simulink model "PMSM_DPCC_NLESO_MRAS"  (R2022a)
settings: Solver=FixedStepDiscrete  StartTime=0.0  StopTime=2  FixedStep=Ts  RelTol=1e-3
InitFcn:
  | Ts = 5e-7;%仿真步长
  | Tpwm = 1e-4;%开关周期
  | Tsample = Tpwm/1;%采样周期/控制周期
  | Tspeed = Tsample;%转速采样周期
  | Pn = 4;%电机极对数
  | Ls = 8.5e-3;%定子电感，采用隐极的，Ld=Lq=Ls
  | Rs = 3;%定子电阻
  | flux = 0.1688;%永磁体磁链
  | Vdc = 311;%直流母线电压
  | iqmax = 20;%额定电流
  | J = 5e-3;%转动惯量
  | B = 2.5e-3;%阻尼系数
  | n_init = 0;%初始转速
  | 
  | %这是DSP内部的控制器参数
  | Ls1 = 1*Ls;%电感参数设置为实际电感
  | Ld1 = Ls1;
  | Lq1 = Ls1;
  | Rs1 = 1*Rs;%电阻参数设置为实际电阻
  | flux1 =1*flux;%磁链参数设置为实际磁链
undefined symbols (not defined in the file): DiscIntNeverNeededParam, magnitude
libraries: simulink x9, slpidlib x2, spsDCVoltageSourceLib x1, spsPermanentMagnetSynchronousMachineLib x1, spsUniversalBridgeLib x1, spspowerguiLib x1
(part 1 of 2)
settings Model: SimulationMode=accelerator  Creator=admin  LastModifiedBy=肖思睿
settings SolverCC: AlgebraicLoopSolver=TrustRegion
settings DataIOCC: ReturnWorkspaceOutputs=off
settings DebuggingCC: UnconnectedInputMsg=warning  UnconnectedOutputMsg=warning  UnconnectedLineMsg=warning  SFMachineParentedDataDiag=warning  ArithmeticOperatorsInVariantConditions=warning
settings SFSimCC: CustomCodeUndefinedFunction=UseInterfaceOnly
settings RTWCC: DLArmComputeVersion=19.05

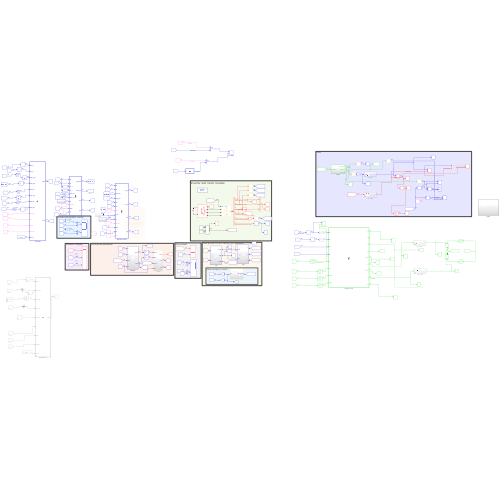
[thumbnail: Simulink's stored preview of the top-level diagram]
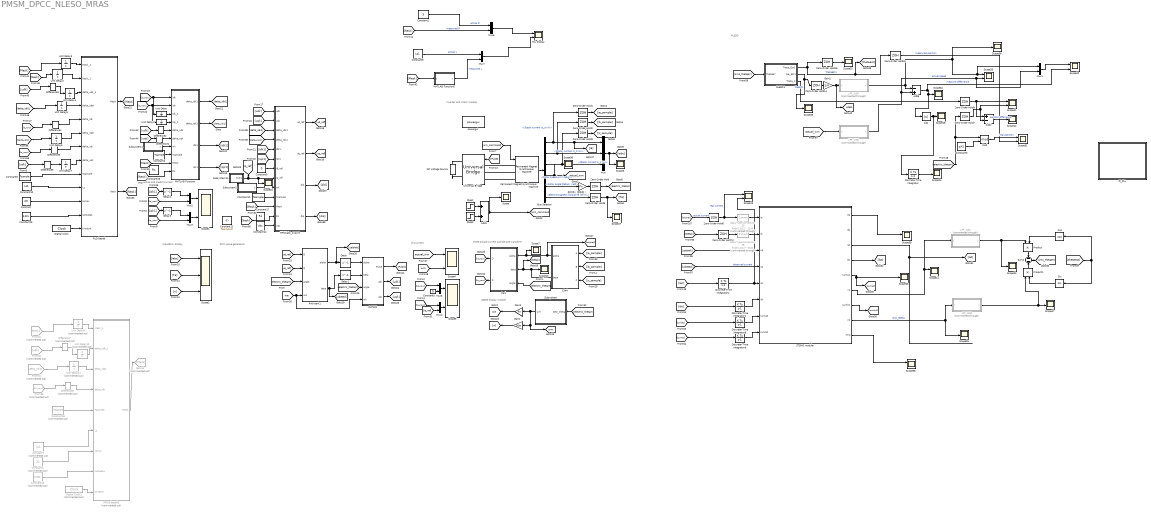
== system PMSM_DPCC_NLESO_MRAS ==
  note: NLESO
  note: PWM pulse generation
  note: Waveform display
  note: actual and predict current
  note: Inverter and motor module
  note: d-q current
  note: three phrase current sample and transform
  note: Speed display module
  Abs : Abs  SaturateOnIntegerOverflow=off
  Add1 : Sum
  Add2 : Sum  Inputs=+-
  Add5 : Sum  Inputs=-+
  Anti-park1 : Subsystem
  Bus Selector : BusSelector  OutputSignals=Stator current is_a (A),Stator current is_b (A),Stator current is_c (A),Rotor speed wm (rad/s),Rotor angle thetam (rad),Electromagnetic torque Te (N*m)
  Clark : Subsystem
  Constant : Constant  Value=20
  Constant1 : Constant  Value=3
  Constant10 : Constant  Value=Ls1
  Constant11 : Constant  Value=Tsample
  Constant12 : Constant  Value=Tpwm/(Ls)
  Constant13 : Constant  Commented=on  Value=0.001
  Constant14 : Constant  Value=Vdc
  Constant15 : Constant  Value=0.001
  Constant16 : Constant  Value=Rs
  Constant17 : Constant  Value=Rs
  Constant18 : Constant  Commented=on  Value=Tsample
  Constant2 : Constant  Value=Tsample
  Constant3 : Constant  Value=pi*2  OutDataTypeStr=double
  Constant4 : Constant  Commented=on  Value=20
  Constant5 : Constant  Value=0
  Constant6 : Constant  Value=Tsample
  Constant7 : Constant  Commented=on  Value=Ls1
  Constant8 : Constant  Value=Ls1
  Constant9 : Constant  Value=0
  Cos : Trigonometry  Operator=cos
  DC Voltage Source : spsDCVoltageSourceLib/DC Voltage Source  Amplitude=Vdc  Measurements=None
  Data Type Conversion25 : DataTypeConversion  Commented=through  OutDataTypeStr=fixdt(1,16,2^-13,0)  SaturateOnIntegerOverflow=off  RndMeth=Floor
  Data Type Conversion26 : DataTypeConversion  Commented=through  OutDataTypeStr=fixdt(1,16,2^-13,0)  SaturateOnIntegerOverflow=off  RndMeth=Floor
  Delay{,1..3} (4 alike) : Delay  DelayLength=1
  Difference{1..6} (6 alike) : simulink/Discrete/Difference  ICPrevInput=0.0  OutMin=[]  OutMax=[]  OutDataType=fixdt(1, 16)  OutScaling=2^-10  DoSatur=off
  Difference7 : simulink/Discrete/Difference  Commented=on  ICPrevInput=0.0  OutMin=[]  OutMax=[]  OutDataType=fixdt(1, 16)  OutScaling=2^-10  DoSatur=off
  Difference8 : simulink/Discrete/Difference  Commented=on  ICPrevInput=0.0  OutMin=[]  OutMax=[]  OutDataType=fixdt(1, 16)  OutScaling=2^-10  DoSatur=off
  Digital Clock : DigitalClock  SampleTime=1e-4
  Digital Clock1 : DigitalClock  Commented=on  SampleTime=1e-4
  Discrete-Time Integrator : DiscreteIntegrator  SampleTime=-1  ICPrevOutput=DiscIntNeverNeededParam  ICPrevScaledInput=DiscIntNeverNeededParam
  Discrete-Time Integrator1 : DiscreteIntegrator  SampleTime=1e-6  ICPrevOutput=DiscIntNeverNeededParam  ICPrevScaledInput=DiscIntNeverNeededParam
  Discrete-Time Integrator2 : DiscreteIntegrator  SampleTime=1e-6  ICPrevOutput=DiscIntNeverNeededParam  ICPrevScaledInput=DiscIntNeverNeededParam
  Discrete-Time Integrator8 : DiscreteIntegrator  gainval=512  SampleTime=1e-6  ICPrevOutput=DiscIntNeverNeededParam  ICPrevScaledInput=DiscIntNeverNeededParam
  Discrete-Time Integrator9 : DiscreteIntegrator  gainval=512  SampleTime=1e-6  ICPrevOutput=DiscIntNeverNeededParam  ICPrevScaledInput=DiscIntNeverNeededParam
  From15 : From  Commented=on  GotoTag=Mesk
  From16 : From  Commented=on  GotoTag=udk
  From34 : From  Commented=on  GotoTag=delta_idk1
  From35 : From  Commented=on  GotoTag=id_now
  Gain1 : Gain  Gain=30/pi
  Gain2 : Gain  Gain=1/4
  Gain3 : Gain  Gain=Pn
  Goto14 : Goto  Commented=on  GotoTag=Mesk
  LPF_WE1 : Subsystem  Commented=through
  LPF_WE2 : Subsystem  Commented=through
  LPF_WE4 : Subsystem  Commented=through
  LPF_WE6 : Subsystem  Commented=through
  MATLAB Function : MATLAB Function  TreatAsAtomicUnit=on
  MATLAB Function5 : MATLAB Function  TreatAsAtomicUnit=on
  MPCCabc_svpwm : MATLAB Function  TreatAsAtomicUnit=on
  MRAS-based1 : MATLAB Function  Commented=on  TreatAsAtomicUnit=on
  Mod : Math  Operator=mod
  Mux : Mux  Inputs=3
  Mux{1..7} (7 alike) : Mux  Inputs=2
  NLESO1 : Subsystem
  PI_PLL : Subsystem
  "Park " : Subsystem
  Permanent Magnet Synchronous Machine : spsPermanentMagnetSynchronousMachineLib/Permanent Magnet Synchronous Machine  NbPhases=3  FluxDistribution=Sinusoidal  RotorType=Round  MechanicalLoad=Torque Tm  PresetModel=No  ShowDetailedParameters=on  MeasurementBus=off  Resistance=Rs  Inductance=8.5e-3  dqInductances=[0.0009262 0.001024]  La=Ls  MachineConstant=Flux linkage established by magnets (V.s)  Flux=flux  VoltageCst=122.4677  TorqueCst=1.0128  Flat=120  Mechanical=[J B Pn 0]  PolePairs=4  InitialConditions=[n_init/60*2*pi,0, 0,0]  InitialConditions5ph=[0 0 0 0 0 0]  RefAngle=Aligned with phase A axis (original Park)  IterativeDiscreteModel=Trapezoidal non iterative  TsBlock=-1  TsPowergui=0
  Product : Product
  Product1 : Product
  R/L display : Scope  NumInputPorts=2
  RLS-based : MATLAB Function  TreatAsAtomicUnit=on
  STSMO module : MATLAB Function  TreatAsAtomicUnit=on
  SVPWM : Subsystem
  Scope{,3,7,10,12,15..17,23..24,26..28,30,32,34..36} (18 alike) : Scope
  Scope{1,4..5,11,13..14,20,31,33,39,56} (11 alike) : Scope  NumInputPorts=2
  Scope2 : Scope  NumInputPorts=3
  Sin : Trigonometry
  Step2 : Step  Time=0  After=0.1  SampleTime=0
  Step3 : Step  After=2.4  SampleTime=0
  Subsystem : Subsystem
  Subsystem1 : Subsystem
  Subsystem11 : Subsystem
  Subsystem2 : Subsystem
  Sum2 : Sum  Inputs=-|-
  Unit Delay : UnitDelay  SampleTime=-1  HasFrameUpgradeWarning=on
  Unit Delay1 : UnitDelay  SampleTime=-1  HasFrameUpgradeWarning=on
  Unit Delay10 : UnitDelay  Commented=on  SampleTime=Tsample  HasFrameUpgradeWarning=on
  Unit Delay11 : UnitDelay  Commented=on  SampleTime=Tsample  HasFrameUpgradeWarning=on
  Unit Delay2 : UnitDelay  InitialCondition=Rs/2  SampleTime=Tsample  HasFrameUpgradeWarning=on
  Unit Delay3 : UnitDelay  InitialCondition=Tpwm/(Ls)  SampleTime=Tsample  HasFrameUpgradeWarning=on
  Unit Delay{4..7} (4 alike) : UnitDelay  SampleTime=Tsample  HasFrameUpgradeWarning=on
  Unit Delay9 : UnitDelay  Commented=on  InitialCondition=Tpwm/(Ls)  SampleTime=Tsample  HasFrameUpgradeWarning=on
  Universal Bridge : spsUniversalBridgeLib/Universal Bridge  Arms=3  SnubberResistance=1e5  SnubberCapacitance=inf  Device=IGBT / Diodes  Ron=1e-3  Lon=0  ForwardVoltages="[  0  0  ]"  ForwardVoltage=0  GTOparameters=[ 10e-6 , 20e-6 ]  IGBTparameters=[ 1e-6 , 2e-6 ]  Measurements=None  Measurements_2=None  converterType=Rectifier
  Zero-Order Hold{,1..3,5} (5 alike) : ZeroOrderHold  SampleTime=Tsample
  Zero-Order Hold{6..7,9..10,14..16} (7 alike) : ZeroOrderHold  SampleTime=1e-4
  powergui : spspowerguiLib/powergui  Priority=1  SimulationMode=Discrete  SampleTime=Ts  frequency=60  Iterations=50  frequencyindice=0  Pbase=100e6  ErrMax=1e-4  UnitsV=kV  UnitsW=MW  buscounter=0  FunctionMessages=off  echomessages=off  EnableUseOfTLC=off  CurrentSourceSwitches=off  DisableSnubberDevices=off  DisableRonSwitches=off  DisableVfSwitches=off  DisplayEquations=off  AutomaticDiscreteSolvers=off  SolverType=Tustin/Backward Euler (TBE)  Interpol=off  ExternalGateDelay=off  methode=off  Ts=100  x0status=blocks  SPID=off  SwTol=0  HookPort=off  NonlinearTolerance=1e-4  nMaxIteration=100  ContinueOnMaxIteration=off  RestoreLinks=warning  ResistiveCurrentMeasurement=off  Frange=[0:2:500]  Ylog=off  Xlog=on  ShowGrid=off  save=off  variable=ZData  structure=IDPCC_MRAS_IA  ZoomFFT=off  StartTime=0  cycles=24  DisplayStyle=1  fundamental=60  FreqAxis=off  MaxFrequency=20000  frequencyindicesteady=1  RmsSteady=1  display=off
  极对数（电角度） : Gain  Gain=Pn
  tag scope: actual_wm=global, wEst=global, we=global, wm=global
  wires:
  Anti-park1/1(alpha) -> [ualphak], Delay/1
  Anti-park1/2(beta) -> Delay1/1, [ubetak]
  [electric_thetam] -> Anti-park1/3(angle)
  Delay/1 -> SVPWM/1(alpha)
  Delay1/1 -> SVPWM/2(beta)
  SVPWM/1(Pulse) -> [Pulse]
  Constant2/1 -> MATLAB Function/8(Tsample)
  [udk] -> Difference2/1
  Difference1/1 -> MATLAB Function/6(delta_uqk)
  Difference2/1 -> MATLAB Function/5(delta_udk)
  Constant14/1 -> MPCCabc_svpwm/13(Vdc)
  [ud_ref] -> Anti-park1/1(D)
  [uq_ref] -> Anti-park1/2(Q)
  [electric_thetam] -> SVPWM/3(angle)
  [iabc] -> Scope2/1
  [n] -> Scope2/3
  [Te] -> Scope2/2
  [idk1] -> Delay2/1
  Mux2/1 -> Scope1/1
  [iqk1] -> Delay3/1
  [id_now] -> Mux2/2
  Mux3/1 -> Scope1/2
  Delay2/1 -> Mux2/1
  [iq_now] -> Mux3/2
  Delay3/1 -> Mux3/1
  MPCCabc_svpwm/1(ud_ref) -> [ud_ref]
  MPCCabc_svpwm/2(uq_ref) -> [uq_ref]
  SVPWM/2(udk) -> [udk]
  SVPWM/3(uqk) -> [uqk]
  Zero-Order Hold3/1 -> [ic_sample]
  Permanent Magnet Synchronous Machine/1 -> Bus Selector/1
  Bus Selector/3 -> Mux/3, Zero-Order Hold3/1  "<Stator current is_c (A)>"
  Bus Selector/2 -> Mux/2, Zero-Order Hold2/1  "<Stator current is_b (A)>"
  极对数（电角度）/1 -> Zero-Order Hold/1
  Bus Selector/5 -> 极对数（电角度）/1  "<Rotor angle thetam (rad)>"
  Bus Selector/4 -> Scope30/1, [actual_wm]  "<Rotor speed wm (rad/s)>"
  Zero-Order Hold5/1 -> Scope27/1, [Te]
  Zero-Order Hold1/1 -> [ia_sample]
  Mux/1 -> Scope3/1, [iabc]
  Bus Selector/6 -> Zero-Order Hold5/1  "<Electromagnetic torque Te (N*m)>"
  [Pulse] -> Universal Bridge/1
  Zero-Order Hold2/1 -> [ib_sample]
  Bus Selector/1 -> [ia], Mux/1, Zero-Order Hold1/1  "<Stator current is_a (A)>"
  "Park "/1(D) -> [id_now]
  Clark/2(beta) -> [ibetak], "Park "/2(beta), Scope10/1
  Gain3/1 -> [we]
  [ia_sample] -> Clark/1(A)
  Gain1/1 -> [n]
  [electric_thetam] -> Subsystem/1(elec_theta)
  "Park "/2(Q) -> [iq_now]
  [ic_sample] -> Clark/3(C)
  Clark/1(alpha) -> [ialphak], Scope7/1, "Park "/1(alpha)
  Subsystem/1(wm) -> [wm], Gain1/1, Gain3/1
  [electric_thetam] -> "Park "/3(angle)
  Mux5/1 -> Scope5/1
  Constant5/1 -> Mux5/2
  [id_now] -> Mux5/1
  [iq_now] -> Mux4/1
  [iq_ref] -> Mux4/2
  [ib_sample] -> Clark/2(B)
  [wm] -> Scope4/2
  Mux4/1 -> Scope5/2
  [actual_wm] -> Scope4/1
  [we] -> Anti-park1/4(we), SVPWM/4(wk)
  Step2/1 -> Add1/1
  Add1/1 -> Scope/1, [wm_command]
  Step3/1 -> Add1/2
  [id_now] -> Unit Delay/1, MATLAB Function/1(idk)
  [iq_now] -> Unit Delay1/1, MATLAB Function/2(iqk)
  Constant11/1 -> MPCCabc_svpwm/10(Tsample)
  Constant9/1 -> MPCCabc_svpwm/7(id_ref)
  Unit Delay/1 -> MATLAB Function/3(idk_1)
  Unit Delay1/1 -> MATLAB Function/4(iqk_1)
  MATLAB Function/4(iqk1) -> [iqk1]
  MATLAB Function/3(idk1) -> [idk1]
  [iqk1] -> MPCCabc_svpwm/6(iqk1)
  [idk1] -> MPCCabc_svpwm/5(idk1)
  MATLAB Function/2(delta_iqk1) -> [delta_iqk1]
  MATLAB Function/1(delta_idk1) -> [delta_idk1]
  [delta_idk1] -> MPCCabc_svpwm/3(delta_idk1)
  [delta_iqk1] -> MPCCabc_svpwm/4(delta_iqk1)
  [udk] -> MPCCabc_svpwm/1(udk)
  [uqk] -> MPCCabc_svpwm/2(uqk)
  Unit Delay3/1 -> RLS-based/1(Mesk_1)
  [Mesk] -> Unit Delay3/1
  [uqk] -> Difference1/1
  [udk] -> Difference3/1
  Unit Delay4/1 -> RLS-based/3(delta_udk_1)
  Difference3/1 -> Unit Delay4/1
  Unit Delay5/1 -> RLS-based/4(delta_idpk)
  [delta_idk1] -> Unit Delay5/1
  [id_now] -> Difference4/1
  Difference4/1 -> RLS-based/5(delta_idk)
  Constant6/1 -> RLS-based/9(Tsample)
  Constant10/1 -> RLS-based/10(Ls)
  Constant/1 -> RLS-based/11(iqmax)
  Constant15/1 -> RLS-based/12(lanbuda1)
  Constant8/1 -> Mux7/1  "actual L"
  [wm_command] -> Permanent Magnet Synchronous Machine/1
  [Mesk] -> MATLAB Function5/1(u)
  Discrete-Time Integrator9/1 -> STSMO module/8(sumb0)
  STSMO module/4(ibt) -> [ibt]
  STSMO module/7(sumb1) -> [sumb1]
  Product1/1 -> Sum2/2
  [ialphak] -> Zero-Order Hold6/1  "actual current"
  [thetaest] -> Cos/1, Sin/1
  Zero-Order Hold10/1 -> Data Type Conversion26/1
  Cos/1 -> Product/2
  Discrete-Time Integrator2/1 -> Scope13/2, STSMO module/5(ial)  "observed current"
  Discrete-Time Integrator8/1 -> STSMO module/7(suma0)
  [ibetak] -> Zero-Order Hold10/1
  Sin/1 -> Product1/2
  STSMO module/3(iat) -> [iat]
  STSMO module/5(suma1) -> [suma1], Scope28/1
  Sum2/1 -> [smo_thetaerr]
  LPF_WE2/1(y) -> Product1/1, Scope17/1
  Discrete-Time Integrator1/1 -> STSMO module/6(ibl)
  Product/1 -> Sum2/1
  Zero-Order Hold/1 -> [electric_thetam]
  LPF_WE1/1(y) -> Product/1, Scope23/1
  Digital Clock/1 -> RLS-based/13(timecnt)
  RLS-based/1(Mesk) -> [Mesk]
  STSMO module/8(x2) -> Scope26/1, LPF_WE2/1(x)  "Obs_Ebeta"
  STSMO module/6(x1) -> Scope14/1, LPF_WE1/1(x)
  Subsystem11/1(Out1) -> Scope15/1, MPCCabc_svpwm/8(iq_ref), [iq_ref]
  MPCCabc_svpwm/4(diq) -> [diq]
  MPCCabc_svpwm/3(did) -> [did]
  STSMO module/9(tmp) -> Scope56/1
  STSMO module/1(ea) -> Scope39/1
  Data Type Conversion25/1 -> STSMO module/1(ia)
  Data Type Conversion26/1 -> STSMO module/2(ib)
  [ualphak] -> STSMO module/3(ua)
  [ubetak] -> STSMO module/4(ub)
  [suma1] -> Discrete-Time Integrator8/1
  [sumb1] -> Discrete-Time Integrator9/1
  [iat] -> Discrete-Time Integrator2/1
  [ibt] -> Discrete-Time Integrator1/1
  Subsystem2/1(y) -> MPCCabc_svpwm/9(wk)
  Subsystem1/1(y) -> MATLAB Function/7(wk)
  [Mesk] -> MATLAB Function/9(Mesk)
  [Mesk] -> MPCCabc_svpwm/11(Mesk)
  Zero-Order Hold6/1 -> Scope13/1, Data Type Conversion25/1  "real current"
  RLS-based/2(Nesk) -> [Nesk]
  [Nesk] -> Unit Delay2/1
  Unit Delay2/1 -> RLS-based/2(Nesk_1)
  Unit Delay6/1 -> RLS-based/6(delta_iqpk)
  [delta_iqk1] -> Unit Delay6/1
  [iq_now] -> Difference5/1
  Difference5/1 -> RLS-based/7(delta_iqk)
  [Nesk] -> MATLAB Function/10(Rs)
  [Nesk] -> MPCCabc_svpwm/12(Rs)
  [udk] -> Difference6/1
  Difference6/1 -> Unit Delay7/1
  Unit Delay7/1 -> RLS-based/8(delta_uqk)
  Constant1/1 -> Mux6/1  "actual R"
  [Nesk] -> Mux6/2  "measured R"
  MATLAB Function5/1(y) -> Mux7/2  "measured L"
  Mux6/1 -> R/L display/1
  Mux7/1 -> R/L display/2
  [actual_wm] -> LPF_WE6/1(x)
  Discrete-Time Integrator/1 -> Scope24/1
  Gain2/1 -> [wEst], LPF_WE4/1(x)
  [smo_thetaerr] -> NLESO1/1(ThetaErr)
  Zero-Order Hold7/1 -> Scope11/2, Add2/2
  Abs/1 -> Scope16/1, Discrete-Time Integrator/1
  LPF_WE4/1(y) -> Add5/1, Mux1/1, Scope33/1, Scope36/1
  NLESO1/3(Theta_2) -> Zero-Order Hold9/1
  Zero-Order Hold14/1 -> Gain2/1
  Constant3/1 -> Mod/2
  NLESO1/2(We_Est1) -> Scope35/1, Zero-Order Hold14/1  "WeEst1"
  Add5/1 -> Scope20/2, Abs/1, Scope34/1  "measure differrence"
  Zero-Order Hold9/1 -> Add2/1, Scope11/1
  Zero-Order Hold15/1 -> Scope31/2  "measured position"
  NLESO1/1(Theta_Est1) -> Zero-Order Hold16/1, Zero-Order Hold15/1, [thetaest]  "ThetaEst1"
  Mod/1 -> Scope31/1  "real position"
  Mux1/1 -> Scope20/1
  LPF_WE6/1(y) -> Mux1/2, Scope33/2, Add5/2  "actual speed"
  Zero-Order Hold16/1 -> Scope32/1
  [electric_thetam] -> Zero-Order Hold7/1, Mod/1
  Add2/1 -> Scope12/1  "position differrence"
  From15/1 -> Unit Delay9/1
  Constant18/1 -> MRAS-based1/5(Tsample)
  From16/1 -> Difference7/1
  Constant4/1 -> MRAS-based1/7(iqmax)
  Constant13/1 -> MRAS-based1/8(lanbuda1)
  Unit Delay9/1 -> MRAS-based1/1(Mesk_1)
  MRAS-based1/1(Mesk) -> Goto14/1
  Digital Clock1/1 -> MRAS-based1/9(timecnt)
  Difference8/1 -> MRAS-based1/4(delta_idk)
  From34/1 -> Unit Delay11/1
  Unit Delay11/1 -> MRAS-based1/3(delta_idpk)
  Difference7/1 -> Unit Delay10/1
  From35/1 -> Difference8/1
  Constant7/1 -> MRAS-based1/6(Ls)
  Unit Delay10/1 -> MRAS-based1/2(delta_udk_1)
  connections:
  Permanent Magnet Synchronous Machine/LConn3 -- Universal Bridge/LConn3
  Permanent Magnet Synchronous Machine/LConn2 -- Universal Bridge/LConn2
  Universal Bridge/RConn1 -- DC Voltage Source/RConn1
  DC Voltage Source/LConn1 -- Universal Bridge/RConn2
  Permanent Magnet Synchronous Machine/LConn1 -- Universal Bridge/LConn1

== system PMSM_DPCC_NLESO_MRAS/Anti-park1 ==
  D : Inport
  Q : Inport  Port=2
  angle : Inport  Port=3
  we : Inport  Port=4
  Constant : Constant  Value=Tpwm
  Constant1 : Constant
  MATLAB Function : MATLAB Function  TreatAsAtomicUnit=on
  alpha : Outport  VectorParamsAs1DForOutWhenUnconnected=off
  beta : Outport  Port=2  VectorParamsAs1DForOutWhenUnconnected=off
  wires:
  D/1 -> MATLAB Function/1(ud)
  Q/1 -> MATLAB Function/2(uq)
  we/1 -> MATLAB Function/3(we)
  Constant/1 -> MATLAB Function/4(Ts)
  angle/1 -> MATLAB Function/5(theta)
  MATLAB Function/2(ub_ref) -> beta/1
  MATLAB Function/1(ua_ref) -> alpha/1
  Constant1/1 -> MATLAB Function/6(Enable)

== system PMSM_DPCC_NLESO_MRAS/Clark ==
  A : Inport
  B : Inport  Port=2
  C : Inport  Port=3
  Fcn1 : Fcn  Expr=sqrt(3)/3*(u(2)-u(3))
  Fcn2 : Fcn  Expr=(2/3)*(u(1)-0.5*u(2)-0.5*u(3))
  Mux2 : Mux  Inputs=3
  alpha : Outport  VectorParamsAs1DForOutWhenUnconnected=off
  beta : Outport  Port=2  VectorParamsAs1DForOutWhenUnconnected=off
  wires:
  C/1 -> Mux2/3
  Fcn2/1 -> alpha/1
  Fcn1/1 -> beta/1
  A/1 -> Mux2/1
  B/1 -> Mux2/2
  Mux2/1 -> Fcn1/1, Fcn2/1

== system PMSM_DPCC_NLESO_MRAS/LPF_WE1 ==
  x : Inport  OutDataTypeStr=double
  Add : Sum
  Add1 : Sum  Inputs=+-
  Constant : Constant  Value=1000e-6  OutDataTypeStr=single
  Delay : Delay  DelayLength=1  SampleTime=1e-6
  Product : Product
  y : Outport
  wires:
  Delay/1 -> Add1/2, Add/2
  x/1 -> Add1/1
  Add/1 -> Delay/1, y/1
  Product/1 -> Add/1
  Add1/1 -> Product/2
  Constant/1 -> Product/1

== system PMSM_DPCC_NLESO_MRAS/LPF_WE2 ==
  x : Inport  OutDataTypeStr=double
  Add : Sum
  Add1 : Sum  Inputs=+-
  Constant : Constant  Value=1000e-6  OutDataTypeStr=single
  Delay : Delay  DelayLength=1  SampleTime=1e-6
  Product : Product
  y : Outport
  wires:
  Delay/1 -> Add1/2, Add/2
  x/1 -> Add1/1
  Add/1 -> Delay/1, y/1
  Product/1 -> Add/1
  Add1/1 -> Product/2
  Constant/1 -> Product/1

== system PMSM_DPCC_NLESO_MRAS/LPF_WE4 ==
  x : Inport  OutDataTypeStr=double
  Add : Sum
  Add1 : Sum  Inputs=+-
  Constant : Constant  Value=20  OutDataTypeStr=single
  Delay : Delay  DelayLength=1  InitialCondition=0  SampleTime=1e-6
  Gain : Gain  Gain=1e-6
  Product : Product
  y : Outport
  wires:
  Delay/1 -> Add1/2, Add/2
  x/1 -> Add1/1
  Add/1 -> Delay/1, y/1
  Product/1 -> Add/1
  Add1/1 -> Product/2
  Constant/1 -> Gain/1
  Gain/1 -> Product/1

== system PMSM_DPCC_NLESO_MRAS/LPF_WE6 ==
  x : Inport  OutDataTypeStr=double
  Add : Sum
  Add1 : Sum  Inputs=+-
  Constant : Constant  Value=2400  OutDataTypeStr=single
  Delay : Delay  DelayLength=1  InitialCondition=20.944  SampleTime=1e-6
  Gain : Gain  Gain=1e-6
  Product : Product
  y : Outport
  wires:
  Delay/1 -> Add1/2, Add/2
  x/1 -> Add1/1
  Add/1 -> Delay/1, y/1
  Product/1 -> Add/1
  Add1/1 -> Product/2
  Constant/1 -> Gain/1
  Gain/1 -> Product/1

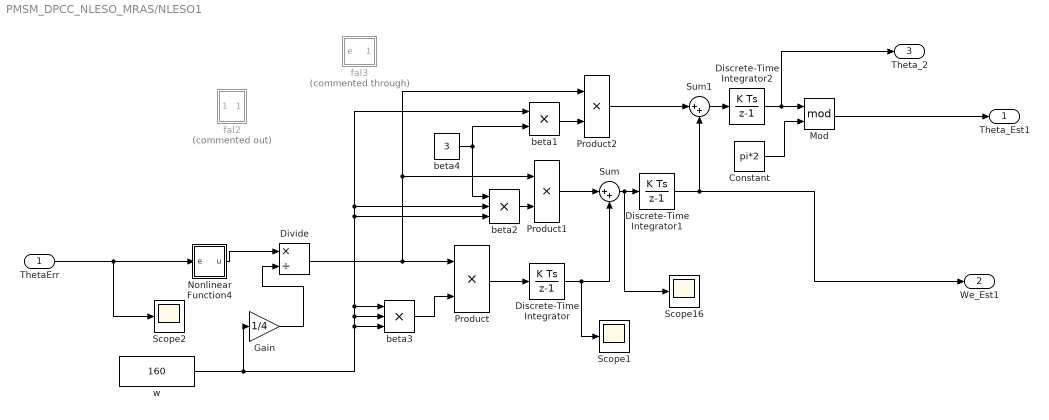
== system PMSM_DPCC_NLESO_MRAS/NLESO1 ==
  ThetaErr : Inport
  Constant : Constant  Value=pi*2  OutDataTypeStr=double
  Discrete-Time Integrator : DiscreteIntegrator  SampleTime=1e-6  ICPrevOutput=DiscIntNeverNeededParam  ICPrevScaledInput=DiscIntNeverNeededParam
  Discrete-Time Integrator1 : DiscreteIntegrator  SampleTime=1e-6  ICPrevOutput=DiscIntNeverNeededParam  ICPrevScaledInput=DiscIntNeverNeededParam
  Discrete-Time Integrator2 : DiscreteIntegrator  SampleTime=1e-6  ICPrevOutput=DiscIntNeverNeededParam  ICPrevScaledInput=DiscIntNeverNeededParam
  Divide : Product  Inputs=*/
  Gain : Gain  Gain=1/4
  Mod : Math  Operator=mod
  Nonlinear Function4 : MATLAB Function  TreatAsAtomicUnit=on
  Product : Product
  Product1 : Product
  Product2 : Product
  Scope1 : Scope
  Scope16 : Scope
  Scope2 : Scope
  Sum : Sum  Inputs=|++
  Sum1 : Sum  Inputs=|++
  beta1 : Product
  beta2 : Product  Inputs=3
  beta3 : Product  Inputs=3
  beta4 : Constant  Value=3  OutDataTypeStr=double
  fal2 : Subsystem  Commented=on  mask{a=1, delta=0.1}
  fal3 : Subsystem  Commented=through  mask{a=0.5, delta=0.05}
  w : Constant  Value=160  OutDataTypeStr=double
  Theta_Est1 : Outport
  We_Est1 : Outport  Port=2
  Theta_2 : Outport  Port=3
  wires:
  Product/1 -> Discrete-Time Integrator/1
  Discrete-Time Integrator/1 -> Scope1/1, Sum/2
  Product1/1 -> Sum/1
  Sum/1 -> Scope16/1, Discrete-Time Integrator1/1
  Product2/1 -> Sum1/1
  Sum1/1 -> Discrete-Time Integrator2/1
  Discrete-Time Integrator2/1 -> Theta_2/1, Mod/1
  Constant/1 -> Mod/2
  Mod/1 -> Theta_Est1/1
  w/1 -> Gain/1, beta2/3, beta2/2, beta1/1, beta3/1, beta3/2, beta3/3
  beta3/1 -> Product/2
  beta1/1 -> Product2/2
  beta4/1 -> beta1/2, beta2/1
  beta2/1 -> Product1/2
  ThetaErr/1 -> Scope2/1, Nonlinear Function4/1(e)
  Discrete-Time Integrator1/1 -> We_Est1/1, Sum1/2
  Nonlinear Function4/1(u) -> Divide/1
  Divide/1 -> Product2/1, Product1/1, Product/1
  Gain/1 -> Divide/2

== system PMSM_DPCC_NLESO_MRAS/PI_PLL ==
  Add4 : Sum  Commented=on  Inputs=+-
  From15 : From  Commented=on  GotoTag=actual_wm  TagVisibility=global
  From66 : From  Commented=on  GotoTag=smo_thetaerr
  Gain5 : Gain  Commented=on  Gain=1/4
  Goto32 : Goto  Commented=on  GotoTag=thetaest
  PLL : Subsystem  Commented=on
  Scope18 : Scope  Commented=on
  Scope19 : Scope  Commented=on  NumInputPorts=2
  Scope21 : Scope  Commented=on
  Zero-Order Hold11 : ZeroOrderHold  Commented=on  SampleTime=Tsample
  Zero-Order Hold8 : ZeroOrderHold  Commented=on  SampleTime=Tsample
  wires:
  From15/1 -> Add4/2, Scope19/2
  Add4/1 -> Scope21/1
  Zero-Order Hold8/1 -> Scope18/1
  PLL/2(Theta_Est) -> Goto32/1, Zero-Order Hold8/1  "ThetaEst"
  From66/1 -> PLL/1(ThetaErr)
  PLL/1(We_Est) -> Zero-Order Hold11/1  "WeEst"
  Gain5/1 -> Add4/1, Scope19/1
  Zero-Order Hold11/1 -> Gain5/1

== system PMSM_DPCC_NLESO_MRAS/Park  ==
  alpha : Inport
  beta : Inport  Port=2
  angle : Inport  Port=3
  Fcn1 : Fcn  Expr=-sin(u(3))*u(1)+cos(u(3))*u(2)
  Fcn2 : Fcn  Expr=cos(u(3))*u(1)+sin(u(3))*u(2)
  Mux2 : Mux  Inputs=3
  D : Outport  VectorParamsAs1DForOutWhenUnconnected=off
  Q : Outport  Port=2  VectorParamsAs1DForOutWhenUnconnected=off
  wires:
  angle/1 -> Mux2/3
  Mux2/1 -> Fcn2/1, Fcn1/1
  Fcn2/1 -> D/1
  Fcn1/1 -> Q/1
  alpha/1 -> Mux2/1
  beta/1 -> Mux2/2

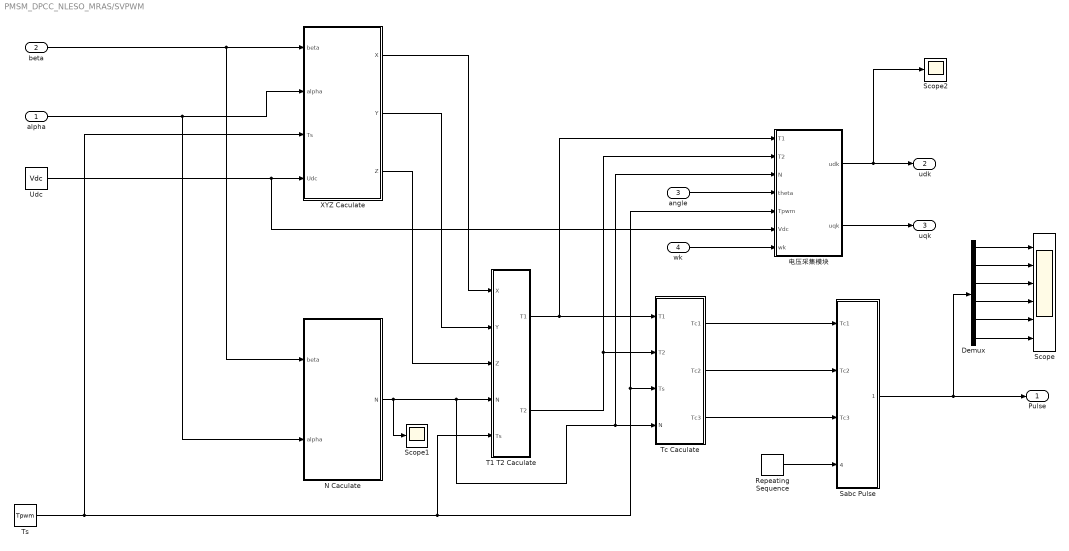
== system PMSM_DPCC_NLESO_MRAS/SVPWM ==
  alpha : Inport
  beta : Inport  Port=2
  angle : Inport  Port=3
  wk : Inport  Port=4
  Demux : Demux  Outputs=6
  N Caculate : Subsystem
  Repeating Sequence : simulink/Sources/Repeating Sequence  rep_seq_t=[0 0.5*Tpwm Tpwm]  rep_seq_y=[0 0.5*Tpwm 0]
  Sabc Pulse : Subsystem
  Scope : Scope  NumInputPorts=6
  Scope1 : Scope
  Scope2 : Scope
  T1 T2 Caculate : Subsystem
  Tc Caculate : Subsystem
  Ts : Constant  Value=Tpwm
  "Udc " : Constant  Value=Vdc
  XYZ Caculate : Subsystem
  电压采集模块 : MATLAB Function  TreatAsAtomicUnit=on
  Pulse : Outport  VectorParamsAs1DForOutWhenUnconnected=off
  udk : Outport  Port=2  VectorParamsAs1DForOutWhenUnconnected=off
  uqk : Outport  Port=3  VectorParamsAs1DForOutWhenUnconnected=off
  wires:
  beta/1 -> N Caculate/1(beta), XYZ Caculate/1(beta)
  alpha/1 -> N Caculate/2(alpha), XYZ Caculate/2(alpha)
  XYZ Caculate/1(X) -> T1 T2 Caculate/1(X)
  XYZ Caculate/2(Y) -> T1 T2 Caculate/2(Y)
  XYZ Caculate/3(Z) -> T1 T2 Caculate/3(Z)
  N Caculate/1(N) -> Scope1/1, 电压采集模块/3(N), Tc Caculate/4(N), T1 T2 Caculate/4(N)
  Ts/1 -> XYZ Caculate/3("Ts "), 电压采集模块/5(Tpwm), Tc Caculate/3(Ts), T1 T2 Caculate/5("Ts ")
  T1 T2 Caculate/1(T1) -> 电压采集模块/1(T1), Tc Caculate/1(T1)
  T1 T2 Caculate/2(T2) -> 电压采集模块/2(T2), Tc Caculate/2(T2)
  Tc Caculate/1(Tc1) -> Sabc Pulse/1(Tc1)
  Tc Caculate/2(Tc2) -> Sabc Pulse/2(Tc2)
  Tc Caculate/3(Tc3) -> Sabc Pulse/3(Tc3)
  Repeating Sequence/1 -> Sabc Pulse/4(Wave)
  angle/1 -> 电压采集模块/4(theta)
  "Udc "/1 -> 电压采集模块/6(Vdc), XYZ Caculate/4(Udc)
  电压采集模块/1(udk) -> Scope2/1, udk/1
  电压采集模块/2(uqk) -> uqk/1
  Sabc Pulse/1("Pulse ") -> Demux/1, Pulse/1
  Demux/4 -> Scope/4
  Demux/5 -> Scope/5
  Demux/3 -> Scope/3
  Demux/2 -> Scope/2
  Demux/6 -> Scope/6
  Demux/1 -> Scope/1
  wk/1 -> 电压采集模块/7(wk)

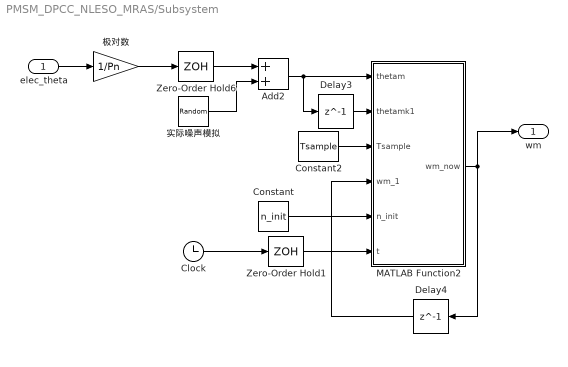
== system PMSM_DPCC_NLESO_MRAS/Subsystem ==
  elec_theta : Inport
  Add2 : Sum
  Clock : Clock
  Constant : Constant  Value=n_init
  Constant2 : Constant  Value=Tsample
  Delay3 : Delay  DelayLength=1
  Delay4 : Delay  DelayLength=1
  MATLAB Function2 : MATLAB Function  TreatAsAtomicUnit=on
  Zero-Order Hold1 : ZeroOrderHold  SampleTime=Tsample
  Zero-Order Hold6 : ZeroOrderHold  SampleTime=Tsample
  实际噪声模拟 : RandomNumber  Mean=0.00000000125  Variance=0.00000000125  SampleTime=Tsample
  极对数 : Gain  Gain=1/Pn
  wm : Outport  VectorParamsAs1DForOutWhenUnconnected=off
  wires:
  MATLAB Function2/1(wm_now) -> wm/1, Delay4/1
  elec_theta/1 -> 极对数/1
  Add2/1 -> Delay3/1, MATLAB Function2/1(thetam)
  Delay4/1 -> MATLAB Function2/4(wm_1)
  极对数/1 -> Zero-Order Hold6/1
  Zero-Order Hold6/1 -> Add2/1
  Delay3/1 -> MATLAB Function2/2(thetamk1)
  Constant2/1 -> MATLAB Function2/3(Tsample)
  实际噪声模拟/1 -> Add2/2
  Constant/1 -> MATLAB Function2/5(n_init)
  Zero-Order Hold1/1 -> MATLAB Function2/6(t)
  Clock/1 -> Zero-Order Hold1/1

== system PMSM_DPCC_NLESO_MRAS/Subsystem1 ==
  Digital Clock : DigitalClock  SampleTime=1e-4
  MATLAB Function3 : MATLAB Function  TreatAsAtomicUnit=on
  Scope : Scope
  y : Outport
  wires:
  [wEst] -> MATLAB Function3/2(wstable)
  [wm] -> MATLAB Function3/1(winit)
  MATLAB Function3/1(y) -> y/1
  Digital Clock/1 -> MATLAB Function3/3(t), Scope/1

== system PMSM_DPCC_NLESO_MRAS/Subsystem11 ==
  Add13 : Sum  Inputs=++-
  Constant22 : Constant  Value=10
  Discrete PID Controller : slpidlib/PID Controller  Controller=PID  Form=Parallel  TimeDomain=Discrete-time  UseExternalTs=off  SampleTime=1e-4  IntegratorMethod=Forward Euler  FilterMethod=Forward Euler  ControllerParametersSource=internal  P=2  I=0.02  UseKiTs=off  D=0  N=100  UseFilter=off  TunerSelectOption=Transfer Function Based (PID Tuner App)  InitialConditionSource=internal  InitialConditionForIntegrator=0  InitialConditionForFilter=0  DifferentiatorICPrevScaledInput=0  ExternalReset=none  TrackingMode=off  Kt=1  LimitOutput=off  SatLimitsSource=internal  UpperSaturationLimit=inf  LowerSaturationLimit=-inf  LinearizeAsGain=off  AntiWindupMode=none  Kb=1  POutMin=[]  POutMax=[]  IOutMin=[]  IOutMax=[]  DOutMin=[]  DOutMax=[]  NOutMin=[]  NOutMax=[]  SumOutMin=[]  SumOutMax=[]  SaturationOutMin=[]  SaturationOutMax=[]  PParamMin=[]  PParamMax=[]  IParamMin=[]  IParamMax=[]  DParamMin=[]  DParamMax=[]  NParamMin=[]  NParamMax=[]  KbParamMin=[]  KbParamMax=[]  KtParamMin=[]  KtParamMax=[]  KbOutMin=[]  KbOutMax=[]  KtOutMin=[]  KtOutMax=[]  IntegratorOutMin=[]  IntegratorOutMax=[]  FilterOutMin=[]  FilterOutMax=[]  SumI1OutMin=[]  SumI1OutMax=[]  SumI2OutMin=[]  SumI2OutMax=[]  SumI3OutMin=[]  SumI3OutMax=[]  SumI4OutMin=[]  SumI4OutMax=[]  SumDOutMin=[]  SumDOutMax=[]  DifferentiatorOutMin=[]  DifferentiatorOutMax=[]  FilterDiffOutCoefMin=[]  FilterDiffOutCoefMax=[]  ReciprocalOutMin=[]  ReciprocalOutMax=[]  SumDenOutMin=[]  SumDenOutMax=[]  SumNumOutMin=[]  SumNumOutMax=[]  DivideOutMin=[]  DivideOutMax=[]  UdiffTsProdOutMin=[]  UdiffTsProdOutMax=[]  NTsProdOutMin=[]  NTsProdOutMax=[]  UintegralTsProdOutMin=[]  UintegralTsProdOutMax=[]  UngainTsProdOutMin=[]  UngainTsProdOutMax=[]  IntegratorContinuousStateAttributes=''  IntegratorStateMustResolveToSignalObject=off  IntegratorRTWStateStorageClass=Auto  FilterContinuousStateAttributes=''  FilterStateMustResolveToSignalObject=off  FilterRTWStateStorageClass=Auto  ParallelPVariant=InternalParameters  IdealPVariant=Disabled  IVariant=InternalParameters  DVariant=InternalParameters  IntegratorVariant=Discrete  SatVariant=Disabled  AWVariant=Passthrough  PCopyVariant=Disabled  TRVariant=Disabled  FdbkBlocksVariant=Forward  IdealPFdbkVariant=Disabled  SatFdbkVariant=Disabled  DerivativeFilterVariant=Differentiator  NVariant=Passthrough  NCopyVariant=Disabled_SignalSpec  FilterICVariant=InternalICsDifferentiator  IntegratorICVariant=InternalICs  ExternalResetVariant=Disabled  TRSumVariant=Passthrough  SumFdbkVariant=Disabled  SumVariant=Sum_PID  TsampFilterVariant=InternalTs  TsampNgainVariant=Passthrough  TsampIntegralVariant=Passthrough  ExternalSaturationOutDataTypeStr=Inherit: Same as second input  aMode=0
  Saturation : Saturate  UpperLimit=8  LowerLimit=-8
  Step4 : Step  Time=0.6  After=120  SampleTime=0
  Subsystem9 : Subsystem
  Zero-Order Hold4 : ZeroOrderHold  SampleTime=Tsample
  Out1 : Outport
  wires:
  Discrete PID Controller/1 -> Saturation/1
  Step4/1 -> Add13/2
  Zero-Order Hold4/1 -> Out1/1
  Constant22/1 -> Add13/1
  Add13/1 -> Discrete PID Controller/1
  Saturation/1 -> Zero-Order Hold4/1
  [actual_wm] -> Add13/3

== system PMSM_DPCC_NLESO_MRAS/Subsystem2 ==
  Digital Clock : DigitalClock  SampleTime=1e-4
  MATLAB Function3 : MATLAB Function  TreatAsAtomicUnit=on
  y : Outport
  wires:
  [wEst] -> MATLAB Function3/2(wstable)
  [wm] -> MATLAB Function3/1(winit)
  MATLAB Function3/1(y) -> y/1
  Digital Clock/1 -> MATLAB Function3/3(t)

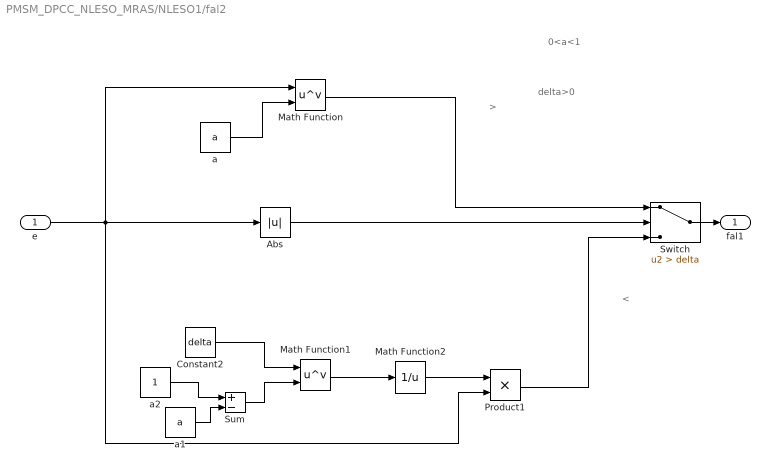
== system PMSM_DPCC_NLESO_MRAS/NLESO1/fal2 ==
  note: >
  note: <
  note: delta>0
  note: 0<a<1
  e : Inport
  Abs : Abs  SaturateOnIntegerOverflow=off
  Constant2 : Constant  Value=delta  OutDataTypeStr=single
  Math Function : Math  Operator=pow  SignedPower=on
  Math Function1 : Math  Operator=pow  SignedPower=on
  Math Function2 : Math  Operator=reciprocal  SignedPower=on
  Product1 : Product
  Sum : Sum  Inputs=+-
  Switch : Switch  Criteria=u2 > Threshold  Threshold=delta  SaturateOnIntegerOverflow=off  InputSameDT=off
  a : Constant  Value=a  OutDataTypeStr=single
  a1 : Constant  Value=a  OutDataTypeStr=single
  a2 : Constant  OutDataTypeStr=single
  fal1 : Outport  VectorParamsAs1DForOutWhenUnconnected=off
  wires:
  Sum/1 -> Math Function1/2
  a1/1 -> Sum/2
  a2/1 -> Sum/1
  Math Function2/1 -> Product1/1
  Abs/1 -> Switch/2
  Math Function/1 -> Switch/1
  Product1/1 -> Switch/3
  Math Function1/1 -> Math Function2/1
  Constant2/1 -> Math Function1/1
  a/1 -> Math Function/2
  e/1 -> Abs/1, Product1/2, Math Function/1
  Switch/1 -> fal1/1

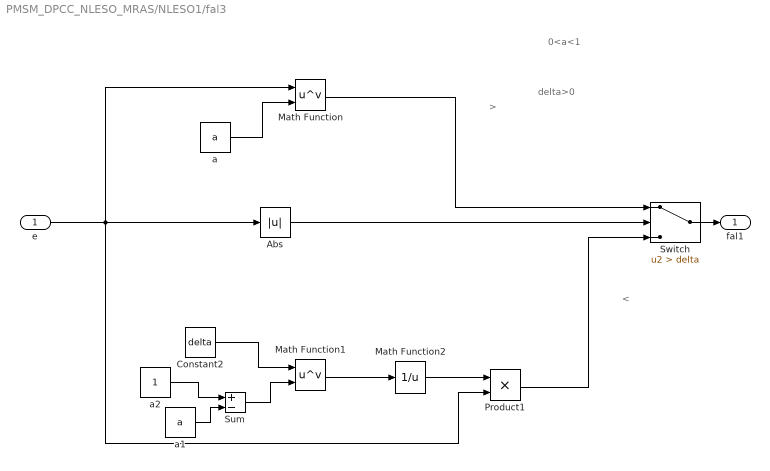
== system PMSM_DPCC_NLESO_MRAS/NLESO1/fal3 ==
  note: 0<a<1
  note: delta>0
  note: <
  note: >
  e : Inport
  Abs : Abs  SaturateOnIntegerOverflow=off
  Constant2 : Constant  Value=delta  OutDataTypeStr=double
  Math Function : Math  Operator=pow  SignedPower=on  OutputSignalType=real
  Math Function1 : Math  Operator=pow  SignedPower=on
  Math Function2 : Math  Operator=reciprocal  SignedPower=on
  Product1 : Product
  Sum : Sum  Inputs=+-
  Switch : Switch  Criteria=u2 > Threshold  Threshold=delta  SaturateOnIntegerOverflow=off  InputSameDT=off
  a : Constant  Value=a  OutDataTypeStr=double
  a1 : Constant  Value=a  OutDataTypeStr=double
  a2 : Constant  OutDataTypeStr=double
  fal1 : Outport  VectorParamsAs1DForOutWhenUnconnected=off
  wires:
  Switch/1 -> fal1/1
  e/1 -> Math Function/1, Product1/2, Abs/1
  a/1 -> Math Function/2
  Constant2/1 -> Math Function1/1
  Math Function1/1 -> Math Function2/1
  Product1/1 -> Switch/3
  Math Function/1 -> Switch/1
  Abs/1 -> Switch/2
  Math Function2/1 -> Product1/1
  a2/1 -> Sum/1
  a1/1 -> Sum/2
  Sum/1 -> Math Function1/2

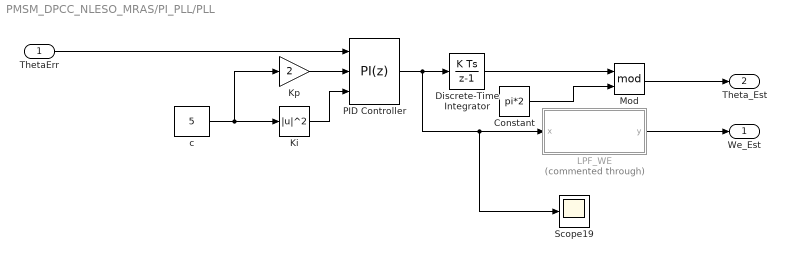
== system PMSM_DPCC_NLESO_MRAS/PI_PLL/PLL ==
  ThetaErr : Inport
  Constant : Constant  Value=pi*2  OutDataTypeStr=double
  Discrete-Time Integrator : DiscreteIntegrator  SampleTime=1e-6  ICPrevOutput=DiscIntNeverNeededParam  ICPrevScaledInput=DiscIntNeverNeededParam
  Ki : Math  Operator=magnitude^2
  Kp : Gain  Gain=2
  LPF_WE : Subsystem  Commented=through
  Mod : Math  Operator=mod
  PID Controller : slpidlib/PID Controller  Controller=PI  Form=Parallel  TimeDomain=Discrete-time  UseExternalTs=off  SampleTime=-1  IntegratorMethod=Forward Euler  FilterMethod=Forward Euler  ControllerParametersSource=external  P=1  I=1  UseKiTs=off  D=0  N=100  UseFilter=on  TunerSelectOption=Transfer Function Based (PID Tuner App)  InitialConditionSource=internal  InitialConditionForIntegrator=0  InitialConditionForFilter=0  DifferentiatorICPrevScaledInput=0  ExternalReset=none  TrackingMode=off  Kt=1  LimitOutput=off  SatLimitsSource=internal  UpperSaturationLimit=inf  LowerSaturationLimit=-inf  LinearizeAsGain=on  AntiWindupMode=none  Kb=1  POutMin=[]  POutMax=[]  IOutMin=[]  IOutMax=[]  DOutMin=[]  DOutMax=[]  NOutMin=[]  NOutMax=[]  SumOutMin=[]  SumOutMax=[]  SaturationOutMin=[]  SaturationOutMax=[]  PParamMin=[]  PParamMax=[]  IParamMin=[]  IParamMax=[]  DParamMin=[]  DParamMax=[]  NParamMin=[]  NParamMax=[]  KbParamMin=[]  KbParamMax=[]  KtParamMin=[]  KtParamMax=[]  KbOutMin=[]  KbOutMax=[]  KtOutMin=[]  KtOutMax=[]  IntegratorOutMin=[]  IntegratorOutMax=[]  FilterOutMin=[]  FilterOutMax=[]  SumI1OutMin=[]  SumI1OutMax=[]  SumI2OutMin=[]  SumI2OutMax=[]  SumI3OutMin=[]  SumI3OutMax=[]  SumI4OutMin=[]  SumI4OutMax=[]  SumDOutMin=[]  SumDOutMax=[]  DifferentiatorOutMin=[]  DifferentiatorOutMax=[]  FilterDiffOutCoefMin=[]  FilterDiffOutCoefMax=[]  ReciprocalOutMin=[]  ReciprocalOutMax=[]  SumDenOutMin=[]  SumDenOutMax=[]  SumNumOutMin=[]  SumNumOutMax=[]  DivideOutMin=[]  DivideOutMax=[]  UdiffTsProdOutMin=[]  UdiffTsProdOutMax=[]  NTsProdOutMin=[]  NTsProdOutMax=[]  UintegralTsProdOutMin=[]  UintegralTsProdOutMax=[]  UngainTsProdOutMin=[]  UngainTsProdOutMax=[]  IntegratorContinuousStateAttributes=''  IntegratorStateMustResolveToSignalObject=off  IntegratorRTWStateStorageClass=Auto  FilterContinuousStateAttributes=''  FilterStateMustResolveToSignalObject=off  FilterRTWStateStorageClass=Auto  ParallelPVariant=ExternalParameters  IdealPVariant=Disabled  IVariant=ExternalParameters  DVariant=Disabled  IntegratorVariant=Discrete  SatVariant=Disabled  AWVariant=Passthrough  PCopyVariant=Disabled  TRVariant=Disabled  FdbkBlocksVariant=Forward  IdealPFdbkVariant=Disabled  SatFdbkVariant=Disabled  DerivativeFilterVariant=Disabled  NVariant=Disabled  NCopyVariant=Disabled_SignalSpec  FilterICVariant=Disabled  IntegratorICVariant=InternalICs  ExternalResetVariant=Disabled  TRSumVariant=Passthrough  SumFdbkVariant=Disabled  SumVariant=Sum_PI  TsampFilterVariant=InternalTs  TsampNgainVariant=Passthrough  TsampIntegralVariant=Passthrough  ExternalSaturationOutDataTypeStr=Inherit: Same as second input  aMode=0
  Scope19 : Scope
  c : Constant  Value=5  OutDataTypeStr=double
  We_Est : Outport
  Theta_Est : Outport  Port=2
  wires:
  Discrete-Time Integrator/1 -> Mod/1
  PID Controller/1 -> Scope19/1, LPF_WE/1(x), Discrete-Time Integrator/1
  LPF_WE/1(y) -> We_Est/1
  Constant/1 -> Mod/2
  ThetaErr/1 -> PID Controller/1
  Mod/1 -> Theta_Est/1
  c/1 -> Ki/1, Kp/1
  Kp/1 -> PID Controller/2
  Ki/1 -> PID Controller/3

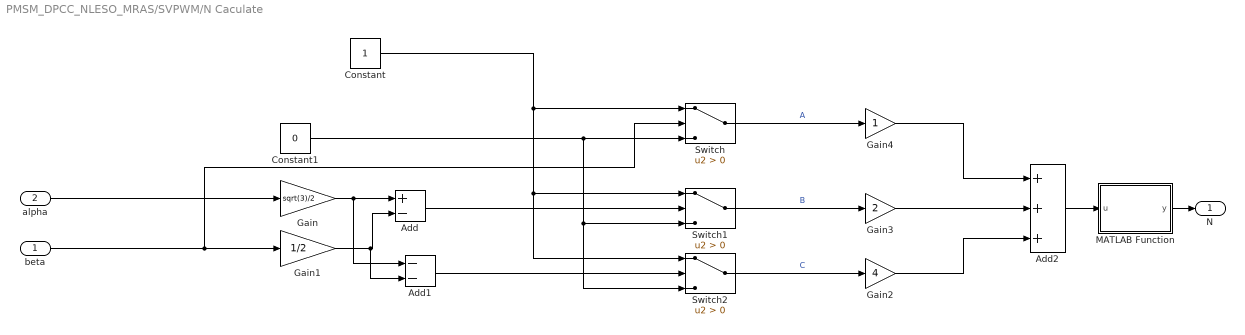
== system PMSM_DPCC_NLESO_MRAS/SVPWM/N Caculate ==
  beta : Inport
  alpha : Inport  Port=2
  Add : Sum  Inputs=+-
  Add1 : Sum  Inputs=--
  Add2 : Sum  Inputs=+++
  Constant : Constant
  Constant1 : Constant  Value=0
  Gain : Gain  Gain=sqrt(3)/2
  Gain1 : Gain  Gain=1/2
  Gain2 : Gain  Gain=4
  Gain3 : Gain  Gain=2
  Gain4 : Gain
  MATLAB Function : MATLAB Function  TreatAsAtomicUnit=on
  Switch : Switch  Criteria=u2 > Threshold  SaturateOnIntegerOverflow=off  InputSameDT=off
  Switch1 : Switch  Criteria=u2 > Threshold  SaturateOnIntegerOverflow=off  InputSameDT=off
  Switch2 : Switch  Criteria=u2 > Threshold  SaturateOnIntegerOverflow=off  InputSameDT=off
  N : Outport  VectorParamsAs1DForOutWhenUnconnected=off
  wires:
  Switch/1 -> Gain4/1  "A"
  Add/1 -> Switch1/2
  Gain/1 -> Add1/1, Add/1
  Gain3/1 -> Add2/2
  Gain2/1 -> Add2/3
  Constant/1 -> Switch/1, Switch2/1, Switch1/1
  Add1/1 -> Switch2/2
  Gain1/1 -> Add1/2, Add/2
  Add2/1 -> MATLAB Function/1(u)
  Constant1/1 -> Switch2/3, Switch1/3, Switch/3
  Gain4/1 -> Add2/1
  beta/1 -> Switch/2, Gain1/1
  Switch2/1 -> Gain2/1  "C"
  Switch1/1 -> Gain3/1  "B"
  alpha/1 -> Gain/1
  MATLAB Function/1(y) -> N/1

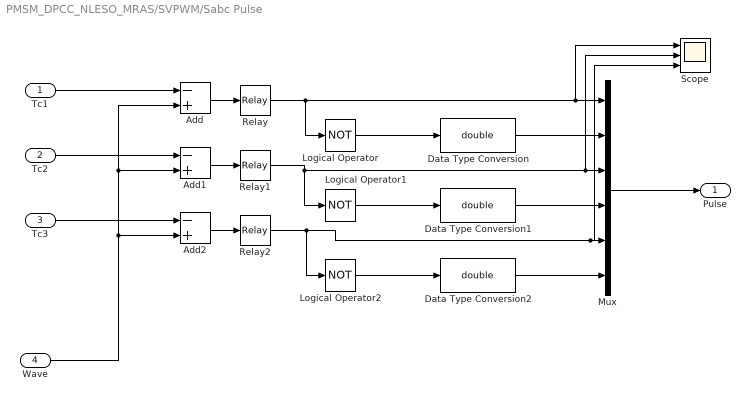
== system PMSM_DPCC_NLESO_MRAS/SVPWM/Sabc Pulse ==
  Tc1 : Inport
  Tc2 : Inport  Port=2
  Tc3 : Inport  Port=3
  Wave : Inport  Port=4
  Add : Sum  Inputs=-+
  Add1 : Sum  Inputs=-+
  Add2 : Sum  Inputs=-+
  Data Type Conversion : DataTypeConversion  OutDataTypeStr=double  SaturateOnIntegerOverflow=off  RndMeth=Floor
  Data Type Conversion1 : DataTypeConversion  OutDataTypeStr=double  SaturateOnIntegerOverflow=off  RndMeth=Floor
  Data Type Conversion2 : DataTypeConversion  OutDataTypeStr=double  SaturateOnIntegerOverflow=off  RndMeth=Floor
  Logical Operator : Logic  Operator=NOT  AllPortsSameDT=off  OutDataTypeStr=boolean
  Logical Operator1 : Logic  Operator=NOT  AllPortsSameDT=off  OutDataTypeStr=boolean
  Logical Operator2 : Logic  Operator=NOT  AllPortsSameDT=off  OutDataTypeStr=boolean
  Mux : Mux  Inputs=6
  Relay : Relay
  Relay1 : Relay
  Relay2 : Relay
  Scope : Scope  NumInputPorts=3
  "Pulse " : Outport  VectorParamsAs1DForOutWhenUnconnected=off
  wires:
  Add/1 -> Relay/1
  Add1/1 -> Relay1/1
  Wave/1 -> Add2/2, Add1/2, Add/2
  Tc2/1 -> Add1/1
  Tc1/1 -> Add/1
  Tc3/1 -> Add2/1
  Logical Operator/1 -> Data Type Conversion/1
  Logical Operator1/1 -> Data Type Conversion1/1
  Add2/1 -> Relay2/1
  Logical Operator2/1 -> Data Type Conversion2/1
  Mux/1 -> "Pulse "/1
  Relay/1 -> Scope/1, Mux/1, Logical Operator/1
  Relay1/1 -> Scope/2, Mux/3, Logical Operator1/1
  Relay2/1 -> Logical Operator2/1, Scope/3, Mux/5
  Data Type Conversion/1 -> Mux/2
  Data Type Conversion1/1 -> Mux/4
  Data Type Conversion2/1 -> Mux/6

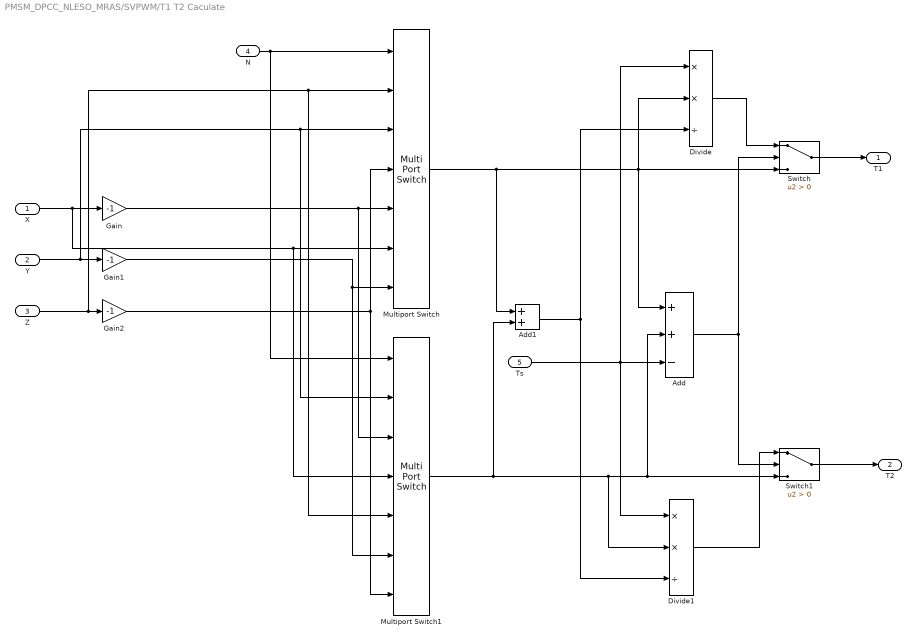
== system PMSM_DPCC_NLESO_MRAS/SVPWM/T1 T2 Caculate ==
  X : Inport
  Y : Inport  Port=2
  Z : Inport  Port=3
  N : Inport  Port=4
  "Ts " : Inport  Port=5
  Add : Sum  Inputs=++-
  Add1 : Sum
  Divide : Product  Inputs=**/
  Divide1 : Product  Inputs=**/
  Gain : Gain  Gain=-1
  Gain1 : Gain  Gain=-1
  Gain2 : Gain  Gain=-1
  Multiport Switch : MultiPortSwitch  Inputs=6  SaturateOnIntegerOverflow=off  InputSameDT=off
  Multiport Switch1 : MultiPortSwitch  Inputs=6  SaturateOnIntegerOverflow=off  InputSameDT=off
  Switch : Switch  Criteria=u2 > Threshold  SaturateOnIntegerOverflow=off  InputSameDT=off
  Switch1 : Switch  Criteria=u2 > Threshold  SaturateOnIntegerOverflow=off  InputSameDT=off
  T1 : Outport  VectorParamsAs1DForOutWhenUnconnected=off
  T2 : Outport  Port=2  VectorParamsAs1DForOutWhenUnconnected=off
  wires:
  Y/1 -> Multiport Switch1/2, Multiport Switch/3, Gain1/1
  X/1 -> Multiport Switch1/4, Multiport Switch/6, Gain/1
  N/1 -> Multiport Switch/1, Multiport Switch1/1
  Z/1 -> Multiport Switch1/5, Multiport Switch/2, Gain2/1
  Gain2/1 -> Multiport Switch1/7, Multiport Switch/4
  Gain/1 -> Multiport Switch1/3, Multiport Switch/5
  Gain1/1 -> Multiport Switch1/6, Multiport Switch/7
  Multiport Switch/1 -> Add1/1, Divide/2, Add/1, Switch/3
  Multiport Switch1/1 -> Add1/2, Divide1/2, Add/2, Switch1/3
  "Ts "/1 -> Divide1/1, Divide/1, Add/3
  Add/1 -> Switch1/2, Switch/2
  Divide/1 -> Switch/1
  Add1/1 -> Divide/3, Divide1/3
  Switch/1 -> T1/1
  Switch1/1 -> T2/1
  Divide1/1 -> Switch1/1

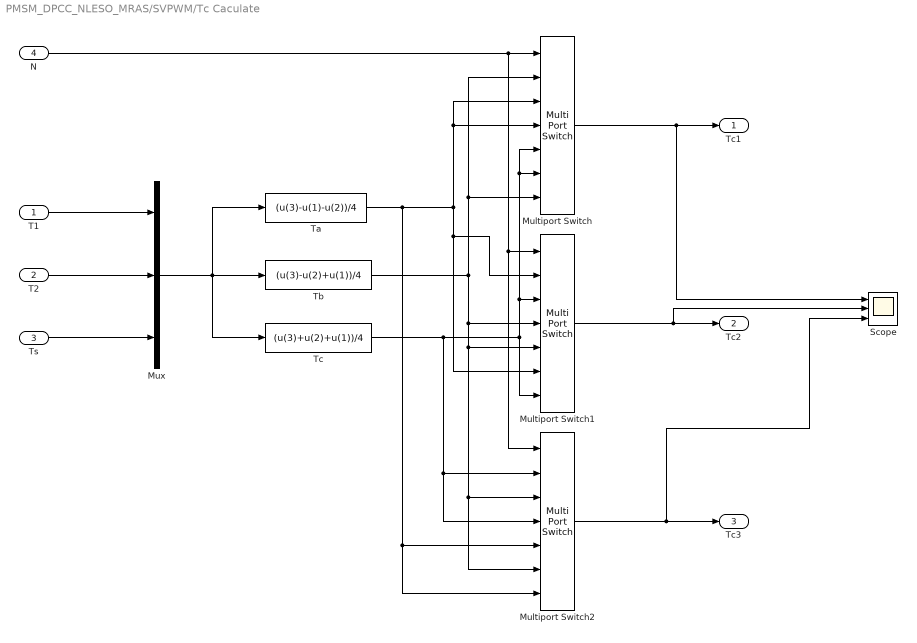
== system PMSM_DPCC_NLESO_MRAS/SVPWM/Tc Caculate ==
  T1 : Inport
  T2 : Inport  Port=2
  Ts : Inport  Port=3
  N : Inport  Port=4
  Multiport Switch : MultiPortSwitch  Inputs=6  SaturateOnIntegerOverflow=off  InputSameDT=off
  Multiport Switch1 : MultiPortSwitch  Inputs=6  SaturateOnIntegerOverflow=off  InputSameDT=off
  Multiport Switch2 : MultiPortSwitch  Inputs=6  SaturateOnIntegerOverflow=off  InputSameDT=off
  Mux : Mux  Inputs=3
  Scope : Scope  NumInputPorts=3
  Ta : Fcn  Expr=(u(3)-u(1)-u(2))/4
  Tb : Fcn  Expr=(u(3)-u(2)+u(1))/4
  Tc : Fcn  Expr=(u(3)+u(2)+u(1))/4
  Tc1 : Outport  VectorParamsAs1DForOutWhenUnconnected=off
  Tc2 : Outport  Port=2  VectorParamsAs1DForOutWhenUnconnected=off
  Tc3 : Outport  Port=3  VectorParamsAs1DForOutWhenUnconnected=off
  wires:
  T2/1 -> Mux/2
  T1/1 -> Mux/1
  Ts/1 -> Mux/3
  Mux/1 -> Tc/1, Ta/1, Tb/1
  N/1 -> Multiport Switch2/1, Multiport Switch1/1, Multiport Switch/1
  Ta/1 -> Multiport Switch2/7, Multiport Switch2/5, Multiport Switch/3, Multiport Switch/4, Multiport Switch1/6, Multiport Switch1/2
  Tb/1 -> Multiport Switch/7, Multiport Switch/2, Multiport Switch1/4, Multiport Switch2/6, Multiport Switch2/3, Multiport Switch1/5
  Tc/1 -> Multiport Switch2/4, Multiport Switch2/2, Multiport Switch1/7, Multiport Switch1/3, Multiport Switch/6, Multiport Switch/5
  Multiport Switch/1 -> Scope/1, Tc1/1
  Multiport Switch1/1 -> Scope/2, Tc2/1
  Multiport Switch2/1 -> Scope/3, Tc3/1

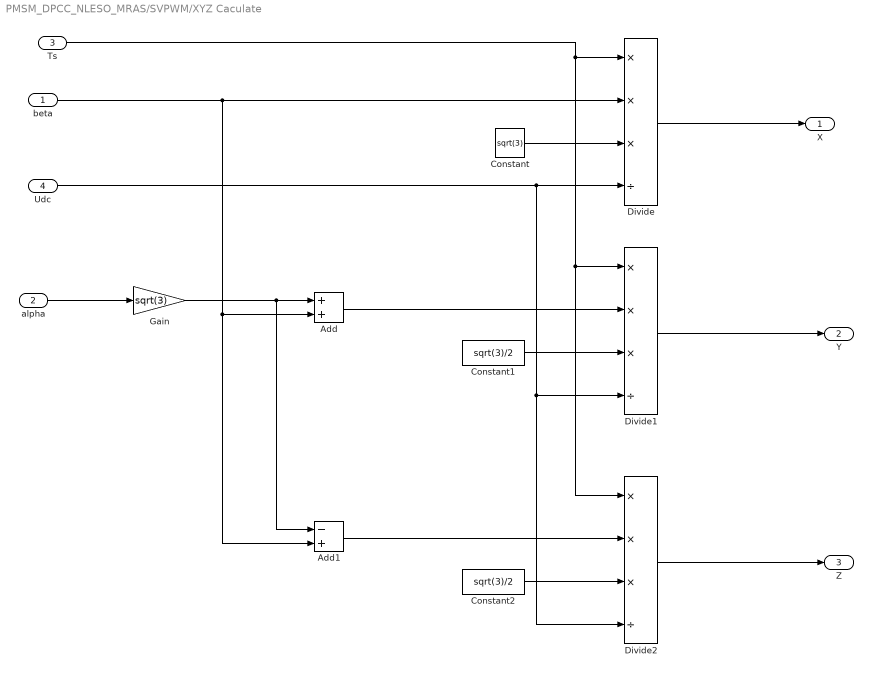
== system PMSM_DPCC_NLESO_MRAS/SVPWM/XYZ Caculate ==
  beta : Inport
  alpha : Inport  Port=2
  "Ts " : Inport  Port=3
  Udc : Inport  Port=4
  Add : Sum
  Add1 : Sum  Inputs=-+
  Constant : Constant  Value=sqrt(3)
  Constant1 : Constant  Value=sqrt(3)/2
  Constant2 : Constant  Value=sqrt(3)/2
  Divide : Product  Inputs=***/
  Divide1 : Product  Inputs=***/
  Divide2 : Product  Inputs=***/
  Gain : Gain  Gain=sqrt(3)
  X : Outport  VectorParamsAs1DForOutWhenUnconnected=off
  Y : Outport  Port=2  VectorParamsAs1DForOutWhenUnconnected=off
  Z : Outport  Port=3  VectorParamsAs1DForOutWhenUnconnected=off
  wires:
  "Ts "/1 -> Divide2/1, Divide1/1, Divide/1
  Udc/1 -> Divide1/4, Divide2/4, Divide/4
  Constant/1 -> Divide/3
  beta/1 -> Add1/2, Add/2, Divide/2
  Constant2/1 -> Divide2/3
  Constant1/1 -> Divide1/3
  Add/1 -> Divide1/2
  Add1/1 -> Divide2/2
  Gain/1 -> Add1/1, Add/1
  alpha/1 -> Gain/1
  Divide1/1 -> Y/1
  Divide/1 -> X/1
  Divide2/1 -> Z/1

== system PMSM_DPCC_NLESO_MRAS/Subsystem11/Subsystem9 ==
  Digital Clock : DigitalClock  SampleTime=1e-4
  MATLAB Function3 : MATLAB Function  TreatAsAtomicUnit=on
  Scope : Scope
  y : Outport
  wires:
  [wEst] -> MATLAB Function3/2(wstable)
  [wm] -> MATLAB Function3/1(winit)
  MATLAB Function3/1(y) -> y/1
  Digital Clock/1 -> MATLAB Function3/3(t), Scope/1

== system PMSM_DPCC_NLESO_MRAS/PI_PLL/PLL/LPF_WE ==
  x : Inport
  Add : Sum
  Add1 : Sum  Inputs=+-
  Constant : Constant  Value=2000  OutDataTypeStr=single
  Delay : Delay  DelayLength=1
  Gain : Gain  Gain=1e-6
  Product : Product
  y : Outport
  wires:
  Delay/1 -> Add1/2, Add/2
  x/1 -> Add1/1
  Add/1 -> Delay/1, y/1
  Product/1 -> Add/1
  Add1/1 -> Product/2
  Constant/1 -> Gain/1
  Gain/1 -> Product/1

== matlab function PMSM_DPCC_NLESO_MRAS/SVPWM/N Caculate/MATLAB Function ==
  data: u input; y output
function y = fcn(u)
if u==0
    y=1;
else
    y = u;
end

== matlab function PMSM_DPCC_NLESO_MRAS/Subsystem/MATLAB Function2 ==
  data: thetam input; wm_now output; thetamk1 input; Tsample input; wm_1 input; n_init input; t input
function wm_now = fcn(thetam,thetamk1,Tsample,wm_1,n_init,t)

wm = (thetam-thetamk1)/Tsample;
    
%离散化低通滤波器的参考网站：
%https://www.zhihu.com/search?type=content&q=%E7%A6%BB%E6%95%A3%E5%8C%96%E4%BD%8E%E9%80%9A%E6%BB%A4%E6%B3%A2%E5%99%A8
%选择低通滤波器截止频率为200Hz，所以可以计算出下列的低通滤波系数
low_pass_factor1 = 2*pi*200*Tsample;
low_pass_factor2 = low_pass_factor1/(1+low_pass_factor1);

%离散化的低通滤波器的表达式
wm_now = low_pass_factor2*wm+(1-low_pass_factor2)*wm_1;

if t==0
    wm_now = n_init/60*2*pi;
end

end

== matlab function PMSM_DPCC_NLESO_MRAS/MRAS-based1 ==
  data: Mesk_1 input; Mesk output; delta_udk_1 input; delta_idpk input; delta_idk input; Tsample input; Ls input; iqmax input; lanbuda1 input; timecnt input
function Mesk   = fcn(Mesk_1,delta_udk_1,delta_idpk,delta_idk,Tsample,Ls,iqmax,lanbuda1,timecnt)
    Ts = Tsample;

    M = Ts/Ls;

    
    ref = 1.5;
    
    Hm = lanbuda1*(iqmax/M)^2*ref;

    
    %    Hn = 1e5;
    %end
% Mesk = M;
    if timecnt == 0.5 %&& timecnt <= 1.2
        Mesk = Ts/(0.6*Ls);

    elseif timecnt == 1.2
        Mesk = Ts/(1.5*Ls);
        
    else
        Mesk = Mesk_1-delta_udk_1*(delta_idpk-delta_idk)/Hm;%fix M
 
    end

   
    

end

== matlab function PMSM_DPCC_NLESO_MRAS/Subsystem1/MATLAB Function3 ==
  data: winit input; y output; wstable input; t input
function y = fcn(winit,wstable,t)
if(t<=5)
    y = winit;
else
    y = wstable;
end

== matlab function PMSM_DPCC_NLESO_MRAS/Subsystem2/MATLAB Function3 ==
  data: winit input; y output; wstable input; t input
function y = fcn(winit,wstable,t)
if(t<5)
    y = winit;
else
    y = wstable;
end

== matlab function PMSM_DPCC_NLESO_MRAS/Subsystem11/Subsystem9/MATLAB Function3 ==
  data: winit input; y output; wstable input; t input
function y = fcn(winit,wstable,t)
if(t<=0.5)
    y = winit;
else
    y = wstable;
end

== matlab function PMSM_DPCC_NLESO_MRAS/Anti-park1/MATLAB Function ==
  data: ud input; ua_ref output; uq input; we input; Ts input; ub_ref output; theta input; Enable input
function [ua_ref,ub_ref] = fcn(ud,uq,we,Ts,theta,Enable)
%这个模块是1.5拍延时补偿环节。
%转速越高的话，在延时对电机的影响越大。

m = we*Ts/(2*sin(0.5*we*Ts));

if (we == 0)||(Enable == 0) %%如果we等于0的话，上面的m无法计算。
   m = 1; 
end

theta_delay = theta+1.5*we*Ts;
ua_ref = m*(cos(theta_delay)*ud - sin(theta_delay)*uq);
ub_ref = m*(sin(theta_delay)*ud + cos(theta_delay)*uq);

end

== matlab function PMSM_DPCC_NLESO_MRAS/MATLAB Function5 ==
  data: u input; y output
function y = fcn(u)

y = 1e-4/u;

== matlab function PMSM_DPCC_NLESO_MRAS/NLESO1/Nonlinear Function4 ==
  data: e input; u output
function u = fcn(e)
a_e = abs(e);
a = 0.5;
dlt = 16;
if a_e <= dlt
    u = e/(dlt^(a-1));
else
    u = sign(e)*a_e^(a);
end

== matlab function PMSM_DPCC_NLESO_MRAS/STSMO module ==
  data: ia input; ib input; ua input; ub input; ea output; eb output; ial input; ibl input; iat output; ibt output; suma0 input; suma1 output; x1 output; sumb0 input; sumb1 output; x2 output; tmp output
function [ea,eb,iat,ibt,suma1,x1,sumb1,x2,tmp] = fcn(ia,ib,ua,ub,ial,ibl,suma0,sumb0)
range = 128;
xia = ial - ia;
xib = ibl - ib;

ea = range*tanh(xia*32);
eb = range*tanh(xib*32);
% if(abs(xia)>0.05)
%     ea = range*sign(xia);
% else
%     ea = range*sin(xia*0.5*pi/0.05);
% end

% ea  = xia*128;
% eb  = xib*128;
% if ea >= range
%     ea = range;
% elseif ea<= -range
%     ea = -range;
% end
% if eb >= range
%     eb = range;
% elseif eb<= -range
%     eb = -range;
% end
% if(abs(xib)>0.05)
%     eb = range*sign(xib);
% else
%     eb = range*sin(xib*0.5*pi/0.55);
% end

suma1 = 1e-6*ea*512;
x1 = 32*sqrt(abs(xia))*ea/2+suma0;
iat = (ua - 3*ia-x1)/0.0085;
sumb1 =  1e-6*eb*512;
x2 = 32*sqrt(abs(xib))*eb/2+sumb0;
tmp = suma1;
ibt = (ub - 3*ib-x2)/0.0085;





end

% iar = ua-0.0085*dia/1e-4-ea;
% ibr = ub-0.0085*dib/1e-4-eb;
% x = atan(-ea/eb);

== matlab function PMSM_DPCC_NLESO_MRAS/MPCCabc_svpwm ==
  data: udk input; uqk input; delta_idk1 input; delta_iqk1 input; idk1 input; ud_ref output; iqk1 input; id_ref input; iq_ref input; wk input; Tsample input; Mesk input; Rs input; uq_ref output; Vdc input; did output; diq output
function [ud_ref,uq_ref,did,diq] = fcn(udk,uqk,delta_idk1,delta_iqk1,idk1,iqk1,id_ref,iq_ref,wk,Tsample,Mesk,Rs,Vdc)
%这个模块的作用就是预测第k+1时刻的所需的电压值
    %ik,uk均应在dq0坐标系下，且为列向量
    Ts=Tsample;
    %Ld=Ls;Lq=Ls;
    A=[1,Ts*wk;
        -Ts*wk,1-Mesk*Rs;];
    B=[Mesk,0;
        0,Mesk;];
    delta_idqk1=[delta_idk1;delta_iqk1];      %转化为列向量
    delta_idqrefk2=[id_ref-idk1;iq_ref-iqk1];      %转化为列向量
    
    B_ni=inv(B);
    delta_udqrefk1=B_ni*(delta_idqrefk2-A*delta_idqk1);
    udrefk1_1 = udk+delta_udqrefk1(1);
    uqrefk1_1 = uqk+delta_udqrefk1(2);
    did = delta_udqrefk1(1);
    diq = delta_udqrefk1(2);
    
    
    %限制Ud的输出不超过电压极限圆
    if  udrefk1_1>(Vdc/sqrt(3))
        udrefk1_1=(Vdc/sqrt(3));
    end
    if  udrefk1_1<=(-Vdc/sqrt(3))
        udrefk1_1=(-Vdc/sqrt(3));
    end
    
    %限制Uq的输出不超过电压极限圆
    if  uqrefk1_1>(Vdc/sqrt(3))
        uqrefk1_1=(Vdc/sqrt(3));
    end
    if  uqrefk1_1<=(-Vdc/sqrt(3))
        uqrefk1_1=(-Vdc/sqrt(3));
    end
    ud_ref = udrefk1_1;
    uq_ref = uqrefk1_1;
    %这是过调制处理

  
end

== matlab function PMSM_DPCC_NLESO_MRAS/MATLAB Function ==
  data: idk input; delta_idk1 output; iqk input; idk_1 input; iqk_1 input; delta_udk input; delta_uqk input; wk input; Tsample input; delta_iqk1 output; Mesk input; Rs input; idk1 output; iqk1 output
function [delta_idk1,delta_iqk1,idk1,iqk1] = fcn(idk,iqk,idk_1,iqk_1,delta_udk,delta_uqk,wk,Tsample,Mesk,Rs)
%这个模块的作用就是预测第k+1时刻的电流
    %ik,uk均应在dq0坐标系下，且为列向量
    Ts=Tsample;
   
    delta_idk=idk-idk_1;
    delta_iqk=iqk-iqk_1;
    A=[1,Ts*wk;
        -Ts*wk,1-Mesk*Rs;];
    B=[Mesk,0;
        0,Mesk;];
    delta_idq0k=[delta_idk;delta_iqk;];      %转化为列向量
    delta_udq0k=[delta_udk;delta_uqk;];      %转化为列向量
    delta_idq0k1=A*delta_idq0k+B*delta_udq0k;       %他也是个3*1列向量
delta_idk1 = delta_idq0k1(1);
delta_iqk1 = delta_idq0k1(2);
idk1=idk+delta_idk1;
iqk1=iqk+delta_iqk1;
end
